simulink model "Longitudinal_Auto_Pilot"  (R2022a)
settings: Solver=VariableStepAuto  StartTime=0.0  StopTime=50  MaxStep=0.001  MinStep=0.00001  RelTol=1e-3
values from neighbouring files (symbols this model uses):
  ath1 = -(1/2/Jy)*rho*(Va^2)*S*c*Cmq*(b/(2*Va))    (= 9.36383713851)    [Long_ctrl.m]
  ath2 = -(1/2/Jy)*rho*(Va^2)*S*c*Cma    (= 53.4084845284)    [Long_ctrl.m]
  ath3 = +(1/2/Jy)*rho*(Va^2)*S*c*Cmde    (= -30.6240015252)    [Long_ctrl.m]
  k_d_teta = (2 * zeta_teta * w_n_teta - ath1) / ath3    [Long_ctrl.m]
  k_i_h = w_n_h^2 / (k_teta_DC * Va)    [Long_ctrl.m]
  k_p_h = 2 * zeta_n_h * w_n_h / (k_teta_DC * Va)    [Long_ctrl.m]
  k_p_teta = delta_e_max * sign(ath3) / error_teta_max    [Long_ctrl.m]
  Va = 10    [Long_ctrl.m]    (also in Variables.m)
settings Model: Creator=Admin  LastModifiedBy=Admin

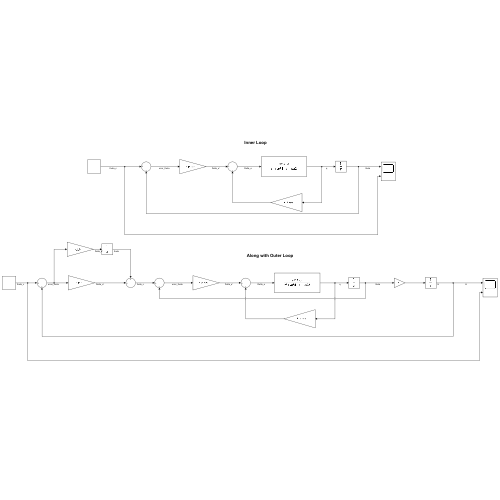
[thumbnail: Simulink's stored preview of the top-level diagram]
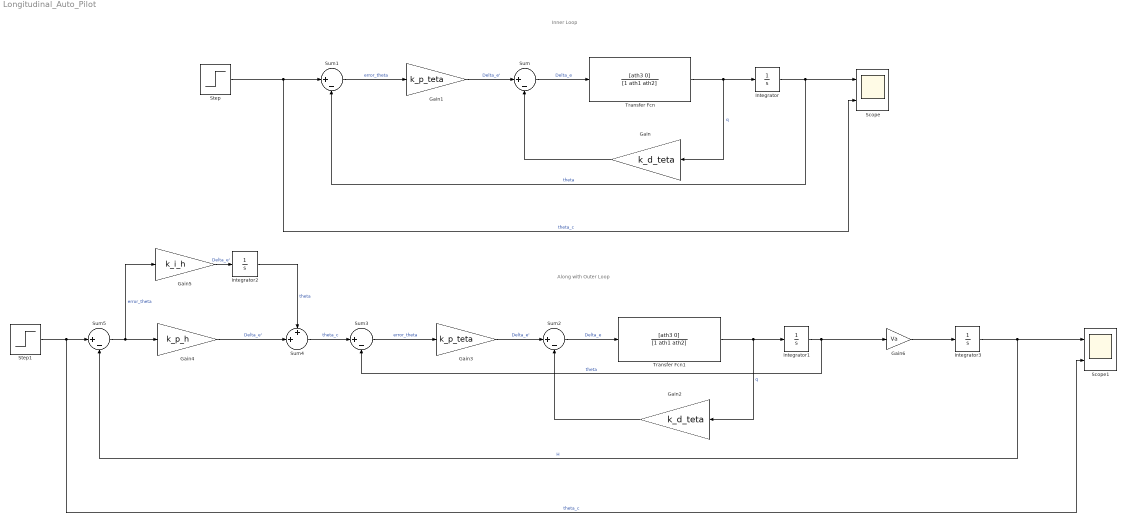
== system Longitudinal_Auto_Pilot ==
  note: Inner Loop
  note: Along with Outer Loop
  Gain : Gain  Gain=k_d_teta
  Gain1 : Gain  Gain=k_p_teta
  Gain2 : Gain  Gain=k_d_teta
  Gain3 : Gain  Gain=k_p_teta
  Gain4 : Gain  Gain=k_p_h
  Gain5 : Gain  Gain=k_i_h
  Gain6 : Gain  Gain=Va
  Integrator{,1..3} (4 alike) : Integrator
  Scope : Scope  NumInputPorts=2
  Scope1 : Scope  NumInputPorts=2
  Step : Step  SampleTime=0
  Step1 : Step  SampleTime=0
  Sum{,1..3,5} (5 alike) : Sum  Inputs=|+-
  Sum4 : Sum  Inputs=++|
  Transfer Fcn : TransferFcn  Numerator=[ath3 0]  Denominator=[1 ath1 ath2]
  Transfer Fcn1 : TransferFcn  Numerator=[ath3 0]  Denominator=[1 ath1 ath2]
  wires:
  Transfer Fcn/1 -> Gain/1, Integrator/1  "q"
  Integrator/1 -> Sum1/2, Scope/1  "theta"
  Gain/1 -> Sum/2
  Sum/1 -> Transfer Fcn/1  "Delta_e"
  Gain1/1 -> Sum/1  "Delta_e'"
  Sum1/1 -> Gain1/1  "error_theta"
  Step/1 -> Scope/2, Sum1/1  "theta_c"
  Sum3/1 -> Gain3/1  "error_theta"
  Gain3/1 -> Sum2/1  "Delta_e'"
  Sum2/1 -> Transfer Fcn1/1  "Delta_e"
  Gain2/1 -> Sum2/2
  Integrator1/1 -> Gain6/1, Sum3/2  "theta"
  Transfer Fcn1/1 -> Integrator1/1, Gain2/1  "q"
  Sum4/1 -> Sum3/1  "theta_c"
  Gain5/1 -> Integrator2/1  "Delta_e'"
  Sum5/1 -> Gain5/1, Gain4/1  "error_theta"
  Gain4/1 -> Sum4/2  "Delta_e'"
  Integrator2/1 -> Sum4/1  "theta"
  Step1/1 -> Scope1/2, Sum5/1  "theta_c"
  Gain6/1 -> Integrator3/1
  Integrator3/1 -> Sum5/2, Scope1/1  "H"
